simulink model "Modele_LQR_6DOF"  (R2025b)
settings: Solver=VariableStepAuto  StartTime=0.0  StopTime=300  FixedStep=0.033333  RelTol=1e-3
values from neighbouring files (symbols this model uses):
  B = -234.459    [AUV_Params.sldd]    (also in block_compute_K.m = [ [                                          0,             )
  Fx1 = -14.142    [AUV_Params.sldd]
  Fx2 = -14.142    [AUV_Params.sldd]
  Fx3 = 0.0    [AUV_Params.sldd]
  Fx4 = 0.0    [AUV_Params.sldd]
  Fx5 = 0.0    [AUV_Params.sldd]
  Fx6 = 0.0    [AUV_Params.sldd]
  Fx7 = 14.142    [AUV_Params.sldd]
  Fx8 = 14.142    [AUV_Params.sldd]
  Fy1 = 14.142    [AUV_Params.sldd]
  Fy2 = -14.142    [AUV_Params.sldd]
  Fy3 = 0.0    [AUV_Params.sldd]
  Fy4 = 0.0    [AUV_Params.sldd]
  Fy5 = 0.0    [AUV_Params.sldd]
  Fy6 = 0.0    [AUV_Params.sldd]
  Fy7 = 14.142    [AUV_Params.sldd]
  Fy8 = -14.142    [AUV_Params.sldd]
  Fz1 = 0.0    [AUV_Params.sldd]
  Fz2 = 0.0    [AUV_Params.sldd]
  Fz3 = -20.0    [AUV_Params.sldd]
  Fz4 = -20.0    [AUV_Params.sldd]
  Fz5 = -20.0    [AUV_Params.sldd]
  Fz6 = -20.0    [AUV_Params.sldd]
  Fz7 = 0.0    [AUV_Params.sldd]
  Fz8 = 0.0    [AUV_Params.sldd]
  I_x = 0.578    [AUV_Params.sldd]
  I_y = 0.645    [AUV_Params.sldd]
  I_z = 0.9366    [AUV_Params.sldd]
  lx1 = 0.0194    [AUV_Params.sldd]
  lx2 = 0.0194    [AUV_Params.sldd]
  lx3 = -0.0317    [AUV_Params.sldd]
  lx4 = -0.0317    [AUV_Params.sldd]
  lx5 = 0.0317    [AUV_Params.sldd]
  lx6 = 0.0317    [AUV_Params.sldd]
  lx7 = -0.0194    [AUV_Params.sldd]
  lx8 = -0.0194    [AUV_Params.sldd]
  ly1 = 0.0381    [AUV_Params.sldd]
  ly2 = -0.0381    [AUV_Params.sldd]
  ly3 = 0.0049    [AUV_Params.sldd]
  ly4 = -0.0049    [AUV_Params.sldd]
  ly5 = 0.0049    [AUV_Params.sldd]
  ly6 = -0.0049    [AUV_Params.sldd]
  ly7 = 0.0381    [AUV_Params.sldd]
  ly8 = -0.0381    [AUV_Params.sldd]
  lz1 = 0.0575    [AUV_Params.sldd]
  lz2 = 0.0575    [AUV_Params.sldd]
  lz3 = 0.0366    [AUV_Params.sldd]
  lz4 = 0.0366    [AUV_Params.sldd]
  lz5 = 0.0366    [AUV_Params.sldd]
  lz6 = 0.0366    [AUV_Params.sldd]
  lz7 = 0.0575    [AUV_Params.sldd]
  lz8 = 0.0575    [AUV_Params.sldd]
  m = 23.9    [AUV_Params.sldd]
  W = 234.459    [AUV_Params.sldd]
  x_rb = 0.0    [AUV_Params.sldd]
  x_rg = 0.0    [AUV_Params.sldd]
  y_rb = 0.0    [AUV_Params.sldd]
  y_rg = 0.0    [AUV_Params.sldd]
  z_rb = 0.0    [AUV_Params.sldd]
  z_rg = 0.0    [AUV_Params.sldd]
undefined symbols (not defined in the file or in its folder): A_num, Q_envoyer, sigbuilder_block, SIZE_TRAJ, T_TRAJ, TRAJECTOIRE, YAW_MODE
libraries: simulink x12, sharedtransform x1, dspinverses x1, SignalEditorBlockLib x1
(part 4 of 4)

== matlab function Modele_LQR_6DOF/Thrustherforces in newtons/MATLAB Function2 ==
  data: u input; tau output
function tau = fcn(u)
%#codegen
lookup =[...
    -40.0337   -1.0000
    -40.0337   -0.9750
    -40.0788   -0.9500
    -37.5428   -0.9250
    -36.6092   -0.9000
    -35.4971   -0.8750
    -33.7623   -0.8500
    -32.3835   -0.8250
    -31.2263   -0.8000
    -29.9809   -0.7750
    -28.5128   -0.7500
    -27.6234   -0.7250
    -26.5554   -0.7000
    -24.7765   -0.6750
    -23.1751   -0.6500
    -22.1522   -0.6250
    -21.3510   -0.6000
    -19.5280   -0.5750
    -18.4600   -0.5500
    -17.3480   -0.5250
    -16.1025   -0.5000
    -14.6345   -0.4750
    -13.0781   -0.4500
    -12.1877   -0.4250
    -10.9874   -0.4000
    -10.0528   -0.3750
    -8.8966   -0.3500
    -7.7404   -0.3250
    -6.8058   -0.3000
    -6.0497   -0.2750
    -5.1151   -0.2500
    -4.2698   -0.2250
    -3.4696   -0.2000
    -2.7135   -0.1750
    -1.8682   -0.1500
    -1.1121   -0.1250
    -0.5335   -0.1000
    -0.2667   -0.0750
    0   -0.0500
    0   -0.0250
    0         0
    0    0.0250
    0    0.0500
    0.5786    0.0750
    1.1121    0.1000
    1.8240    0.1250
    2.5801    0.1500
    3.4255    0.1750
    4.0923    0.2000
    5.1151    0.2250
    6.2272    0.2500
    7.0284    0.2750
    8.2739    0.3000
    9.2526    0.3250
    10.8089    0.3500
    12.2328    0.3750
    13.6558    0.4000
    14.9904    0.4250
    16.4585    0.4500
    17.7039    0.4750
    19.2161    0.5000
    20.5508    0.5250
    21.7521    0.5500
    23.6644    0.5750
    24.7324    0.6000
    26.4221    0.6250
    27.7126    0.6500
    29.6249    0.6750
    31.3156    0.7000
    32.8729    0.7250
    33.8065    0.7500
    34.2517    0.7750
    37.0534    0.8000
    38.6549    0.8250
    39.2776    0.8500
    41.1458    0.8750
    42.9257    0.9000
    44.7938    0.9250
    47.1062    0.9500
    48.0408    0.9750
    49.9531    1.0000];
%Thrustherforce in newtons.
tau = zeros(8,1);
tau(1) = interp1(lookup(:,2),lookup(:,1),u(1));
tau(2) = interp1(lookup(:,2),lookup(:,1),u(2));
tau(3) = interp1(lookup(:,2),lookup(:,1),u(3));
tau(4) = interp1(lookup(:,2),lookup(:,1),u(4));
tau(5) = interp1(lookup(:,2),lookup(:,1),u(5));
tau(6) = interp1(lookup(:,2),lookup(:,1),u(6));
tau(7) = interp1(lookup(:,2),lookup(:,1),u(7));
tau(8) = interp1(lookup(:,2),lookup(:,1),u(8));

end
